simulink model "WT_model"  (R2015a)
settings: Solver=ode3  StartTime=0.0  StopTime=2  FixedStep=Ts  RelTol=1e-3
values from neighbouring files (symbols this model uses):
  radps2rpm = 30/pi    (= 9.54929658551)    [VOC_param.m]    (also in VOC_param_paper.m; power_control_param.m)
  rpm2radps = pi/30    (= 0.10471975512)    [VOC_param.m]    (also in VOC_param_paper.m; power_control_param.m)
  wm2we = p    (= 4)    [VOC_param.m]    (also in VOC_param_paper.m; power_control_param.m)
libraries: powerlib x9
settings Model: Creator=rblan  LastModifiedBy=rblan

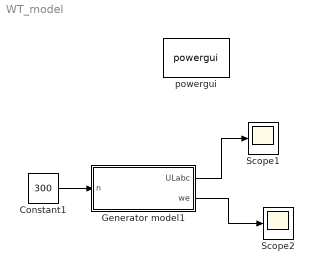
== system WT_model ==
  Constant1 : Constant  Value=300
  Generator model1 : Subsystem
  Scope1 : Scope
      settings: YMin=-400  YMax=400  SaveName=ScopeData3
  Scope2 : Scope
      settings: YMin=-400  YMax=400  SaveName=ScopeData4
  powergui : powerlib/powergui  Priority=1  SimulationMode=Continuous  SolverType=Tustin/Backward Euler (TBE)  SampleTime=50e-6  frequency=60  SPID=off  DisableSnubberDevices=off  DisableRonSwitches=off  DisableVfSwitches=off  SwTol=0  DisplayEquations=off  Interpol=off  methode=off  Ts=100  FunctionMessages=off  echomessages=off  HookPort=off  EnableUseOfTLC=off  x0status=blocks  frequencyindice=0  Pbase=100e6  ErrMax=1e-4  Iterations=50  UnitsV=kV  UnitsW=MW  buscounter=0  RestoreLinks=warning  ResistiveCurrentMeasurement=off  Frange=[0:2:500]  Ylog=off  Xlog=on  ShowGrid=off  save=off  variable=ZData  structure=0  ZoomFFT=off  StartTime=0.0  cycles=1  DisplayStyle=1  fundamental=60  FreqAxis=off  MaxFrequency=1000  frequencyindicesteady=1  RmsSteady=1  display=off
  wires:
  Generator model1/1(ULabc) -> Scope1/1
  Constant1/1 -> Generator model1/1(n)
  Generator model1/2(we) -> Scope2/1

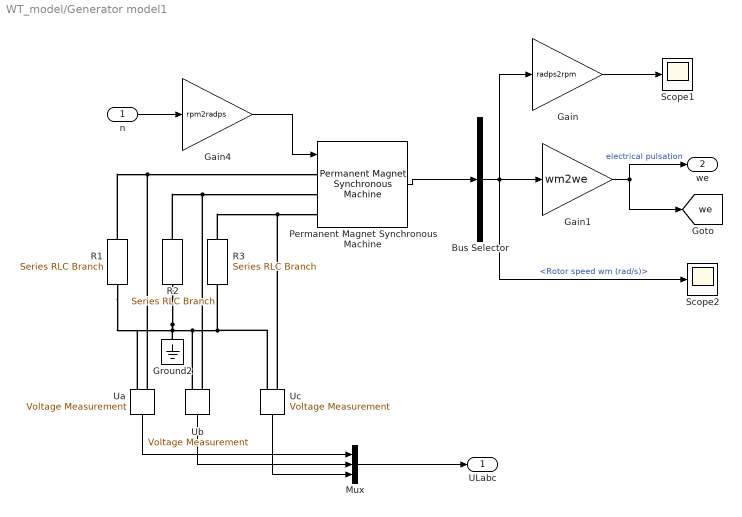
== system WT_model/Generator model1 ==
  n : Inport
  Bus Selector : BusSelector  OutputSignals=Rotor speed wm (rad/s)
  Gain : Gain  Gain=radps2rpm
  Gain1 : Gain  Gain=wm2we
  Gain4 : Gain  Gain=rpm2radps
  Ground2 : powerlib/Elements/Ground  LConnTagsString=a
  Mux : Mux  Inputs=3
  Permanent Magnet Synchronous Machine : powerlib/Machines/Permanent Magnet Synchronous Machine  NbPhases=3  FluxDistribution=Sinusoidal  RotorType=Round  MechanicalLoad=Speed w  PresetModel="07:  20 Nm 300 Vdc 2200 RPM - 33.9 Nm"  ShowDetailedParameters=on  MeasurementBus=off  Resistance=0.129  Inductance=8.5e-3  dqInductances=[8.5e-3,8.5e-3]  La=0.00153  MachineConstant=Flux linkage established by magnets (V.s)  Flux=0.1821  VoltageCst=132.1171  TorqueCst=1.0926  Flat=120  Mechanical=[0.003334 0.000425 4 0]  PolePairs=4  InitialConditions=[0,0, 0,0]  InitialConditions5ph=[0 0 0 0 0 0]  TsPowergui=0  TsBlock=-1  RefAngle=90 degrees behind phase A axis (modified Park)
  R1 : powerlib/Elements/Series RLC Branch  LConnTagsString=__new0  RConnTagsString=__new0  BranchType=R  Resistance=5.6566e-2  Inductance=[]  SetiL0=off  InitialCurrent=0  Capacitance=[]  Setx0=off  InitialVoltage=0  Measurements=None
  R2 : powerlib/Elements/Series RLC Branch  LConnTagsString=__new0  RConnTagsString=__new0  BranchType=R  Resistance=5.6566e-2  Inductance=[]  SetiL0=off  InitialCurrent=0  Capacitance=[]  Setx0=off  InitialVoltage=0  Measurements=None
  R3 : powerlib/Elements/Series RLC Branch  LConnTagsString=__new0  RConnTagsString=__new0  BranchType=R  Resistance=5.6566e-2  Inductance=[]  SetiL0=off  InitialCurrent=0  Capacitance=[]  Setx0=off  InitialVoltage=0  Measurements=None
  Scope1 : Scope
      settings: YMin=2196.34  YMax=2196.34
  Scope2 : Scope
      settings: SaveName=ScopeData2
  Ua : powerlib/Measurements/Voltage Measurement  Tag=PoWeRsYsTeMmEaSuReMeNt  PhasorSimulation=off  OutputType=Magnitude  PSBequivalent=0
  Ub : powerlib/Measurements/Voltage Measurement  Tag=PoWeRsYsTeMmEaSuReMeNt  PhasorSimulation=off  OutputType=Magnitude  PSBequivalent=0
  Uc : powerlib/Measurements/Voltage Measurement  Tag=PoWeRsYsTeMmEaSuReMeNt  PhasorSimulation=off  OutputType=Magnitude  PSBequivalent=0
  ULabc : Outport
  we : Outport  Port=2
  tag scope: we=global
  wires:
  Permanent Magnet Synchronous Machine/1 -> Bus Selector/1
  Bus Selector/1 -> Gain/1, Gain1/1, Scope2/1  "<Rotor speed wm (rad/s)>"
  Ub/1 -> Mux/2
  Mux/1 -> ULabc/1
  Ua/1 -> Mux/1
  Uc/1 -> Mux/3
  Gain/1 -> Scope1/1
  n/1 -> Gain4/1
  Gain4/1 -> Permanent Magnet Synchronous Machine/1
  Gain1/1 -> [we], we/1  "electrical pulsation"
  connections:
  R1/RConn1 -- Ua/LConn1 -- Permanent Magnet Synchronous Machine/LConn1
  R2/RConn1 -- Ub/LConn1 -- Permanent Magnet Synchronous Machine/LConn2
  R3/RConn1 -- Permanent Magnet Synchronous Machine/LConn3 -- Uc/LConn1
  Ground2/LConn1 -- R1/LConn1 -- Ua/LConn2 -- Ub/LConn2 -- Uc/LConn2 -- R3/LConn1 -- R2/LConn1
